simulink model "attitudeModel"  (R2018b)
settings: Solver=VariableStepAuto  StartTime=0.0  StopTime=60  RelTol=1e-3
undefined symbols (not defined in the file or in its folder): fgc
settings Model: Creator=cjmul  LastModifiedBy=cjmul

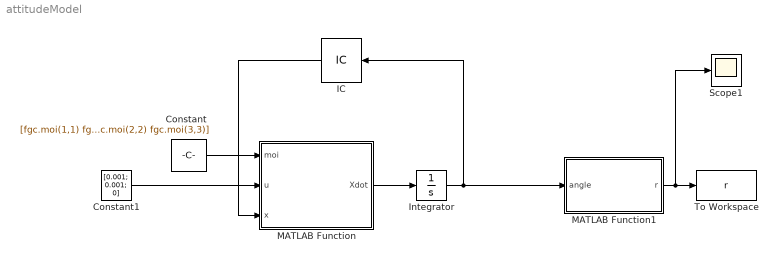
== system attitudeModel ==
  Constant : Constant  Value=[fgc.moi(1,1) fgc.moi(2,2) fgc.moi(3,3)]
  Constant1 : Constant  Value=[0.001; 0.001; 0]
  IC : InitialCondition  Value=[0; 10*pi/180; 0; 0; 0; 0]
  Integrator : Integrator
  MATLAB Function : MATLAB Function  TreatAsAtomicUnit=on
  MATLAB Function1 : MATLAB Function  TreatAsAtomicUnit=on
  Scope1 : Scope
  To Workspace : ToWorkspace  VariableName=r  SaveFormat=Timeseries  SampleTime=-1
  wires:
  Constant/1 -> MATLAB Function/1(moi)
  Integrator/1 -> MATLAB Function1/1(angle), IC/1
  MATLAB Function/1(Xdot) -> Integrator/1
  MATLAB Function1/1(r) -> Scope1/1, To Workspace/1
  Constant1/1 -> MATLAB Function/2(u)
  IC/1 -> MATLAB Function/3(x)

== matlab function attitudeModel/MATLAB Function1 ==
  data: angle input; r output
function r = pointingVector(angle)
        theta   = angle(1);
        phi     = angle(2);
        psi     = angle(3);

        Ry= [cos(theta)     0       sin(theta);
                0           1           0;
             -sin(theta)    0      cos(theta)];

        Rx = [  1           0           0;
                0       cos(phi)    -sin(phi);
                0       sin(phi)    cos(phi)];

        Rz = [cos(psi)  -sin(psi)       0;
              sin(psi)  cos(psi)        0;
                0           0           1];

        rvec = Rz*Ry*Rx*[1;1;1];
        r = rvec/norm(rvec);
end

== matlab function attitudeModel/MATLAB Function ==
  data: moi input; u input; x input; Xdot output
function Xdot = att_dynamics(moi,u,x)
Xdot = zeros(6,1);

Ix = moi(1);
Iy = moi(2);
Iz = moi(3);

Xdot(1,1) = x(4)*cos(x(3))-x(5)*sin(x(3));
Xdot(2,1) = x(4)*sin(x(3))+x(5)*cos(x(3));
Xdot(3,1) = (-x(4)*cos(x(3))+x(5)*sin(x(3)))*tan(x(2))+x(6);
Xdot(4,1) = (Iy-Iz)/Ix*x(5)*x(6)+u(1);
Xdot(5,1) = (Iz-Ix)/Iy*x(6)*x(4)+u(2);
Xdot(6,1) = (Ix-Iy)/Iz*x(4)*x(5)+u(3);

end
